simulink model "plantMRUE2"  (R2023b)
settings: Solver=VariableStepAuto  StartTime=0.0  StopTime=7  RelTol=1e-3
model workspace (MATLAB code in the model file):
  | %% True Parameters
  | % Masses
  | mw=0.1;
  | mb=1;
  | M=1.2;
  | 
  | % Distances
  | rho=0.07;
  | l=0.02;
  | d=0.015; % distance A-C
  | 
  | % Electriques
  | L=1e-3;
  | R=1e-1;
  | % r;
  | 
  | % Couples
  | k=1e-2;
  | % alpha=34.6;
  | % beta=2.06e5;
  | 
  | % Moments inertie
  | Iwy=2.45e-4;
  | Ipsi=1.53e-2;
  | 
  | % Utilitaire
  | beta = (M + 2*Iwy/rho^2);
  | gamma = Ipsi + mb*d^2;
  | 
  | %% Nominal Equilibrium Trajectory: Horizontal MRU
  | 
  | % We command speed
  | uref = 1; %m/s
  | psiref = 0;
  | 
  | Usbar = min([2*k/rho*uref; 12]); % should not be >12V
  | 
  | Urbar = Usbar/2; %right
  | Ulbar = Usbar/2;
  | 
  | pbar = 0; % is not in state function, any value fits
  | % normally, should equals ubar*t.
  | ubar = uref;
  | psibar = psiref;
  | vbar = 0;
  | irbar = 0;
  | ilbar = 0;
  | xbar = pbar;
  | ybar = 0;
  | 
  | % IMPORTANT: following only true at t=0s.
  | statebar = [pbar; ubar; psibar; vbar; irbar; ilbar; xbar; ybar];
settings Model: Creator=Jules  LastModifiedBy=Jules

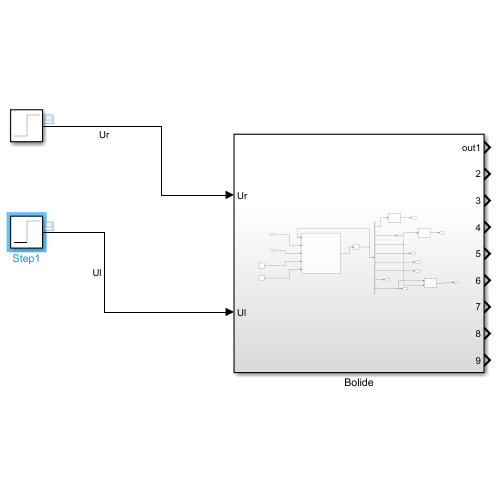
[thumbnail: Simulink's stored preview of the top-level diagram]
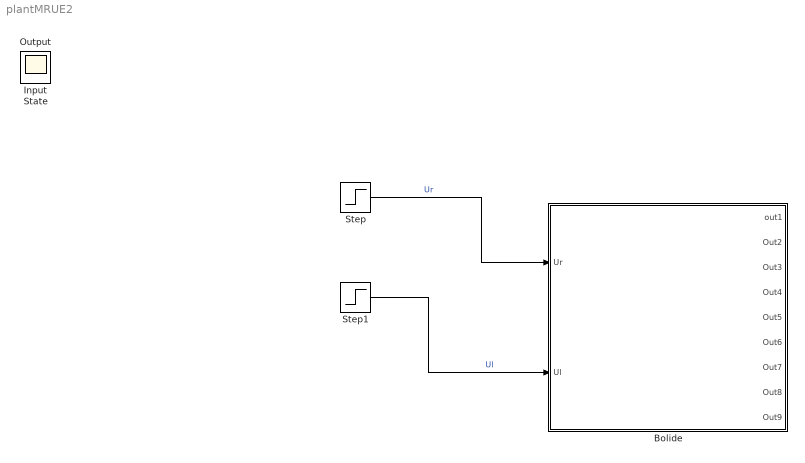
== system plantMRUE2 ==
  Bolide : Subsystem
  Step : Step  Time=5  Before=Urbar  After=Urbar  SampleTime=0
  Step1 : Step  Time=2  Before=Ulbar  After=Ulbar  SampleTime=0
  Input : Scope
  Output : Scope
  State : Scope
  wires:
  Step/1 -> Bolide/1(Ur)  "Ur"
  Step1/1 -> Bolide/2(Ul)  "Ul"

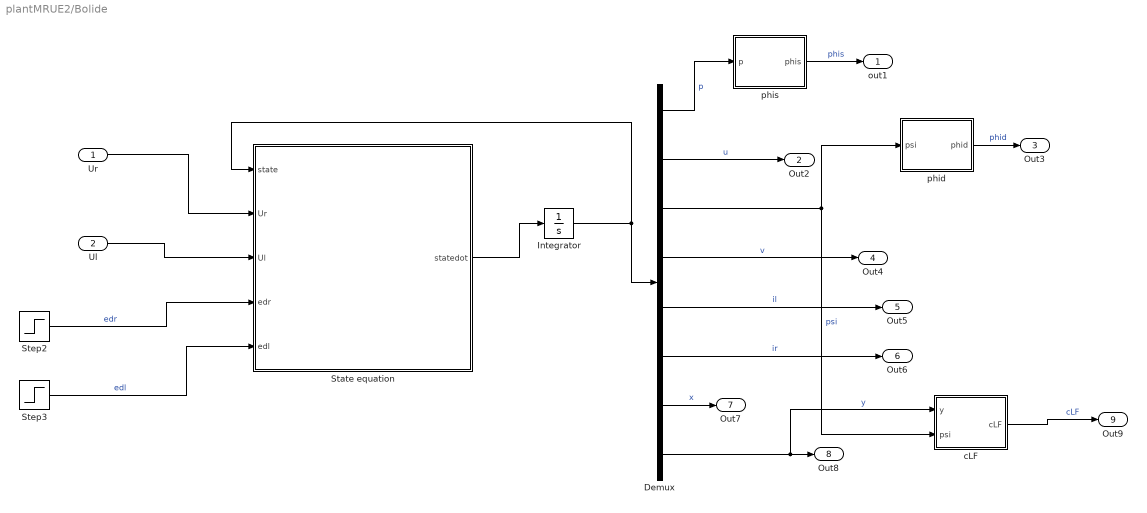
== system plantMRUE2/Bolide ==
  Ur : Inport
  Ul : Inport  Port=2
  Demux : Demux  Outputs=8
  Integrator : Integrator  InitialCondition=statebar
  State equation : MATLAB Function  TreatAsAtomicUnit=on
  Step2 : Step  After=0  SampleTime=0
  Step3 : Step  After=0  SampleTime=0
  cLF : MATLAB Function  TreatAsAtomicUnit=on
  phid : MATLAB Function  TreatAsAtomicUnit=on
  phis : MATLAB Function  TreatAsAtomicUnit=on
  out1 : Outport
  Out2 : Outport  Port=2
  Out3 : Outport  Port=3
  Out4 : Outport  Port=4
  Out5 : Outport  Port=5
  Out6 : Outport  Port=6
  Out7 : Outport  Port=7
  Out8 : Outport  Port=8
  Out9 : Outport  Port=9
  wires:
  Step3/1 -> State equation/5(edl)  "edl"
  State equation/1(statedot) -> Integrator/1
  Integrator/1 -> State equation/1(state), Demux/1
  Step2/1 -> State equation/4(edr)  "edr"
  Ul/1 -> State equation/3(Ul)
  Ur/1 -> State equation/2(Ur)
  Demux/1 -> phis/1(p)  "p"
  Demux/8 -> cLF/1(y), Out8/1  "y"
  Demux/7 -> Out7/1  "x"
  Demux/2 -> Out2/1  "u"
  Demux/6 -> Out6/1  "ir"
  Demux/4 -> Out4/1  "v"
  Demux/5 -> Out5/1  "il"
  phis/1(phis) -> out1/1  "phis"
  Demux/3 -> phid/1(psi), cLF/2(psi)  "psi"
  phid/1(phid) -> Out3/1  "phid"
  cLF/1(cLF) -> Out9/1  "cLF"

== matlab function plantMRUE2/Bolide/cLF ==
  data: y input; cLF output; psi input; psibar parameter; ybar parameter
function cLF = fcn(y, psi, psibar, ybar)

cLF = y/cos(psi - psibar);

== matlab function plantMRUE2/Bolide/State equation ==
  data: state input; statedot output; Ur input; Ul input; edr input; edl input; M parameter; rho parameter; l parameter; Iwy parameter; Ipsi parameter; d parameter; L parameter; R parameter; k parameter; mb parameter; beta parameter; gamma parameter
function statedot = fcn(state,Ur, Ul, edr, edl, M, rho, l, Iwy, Ipsi, d, L, R, k, mb, beta, gamma)
% ed est l'entrée de perturbation, != d (distance AC)
% Model parameters M,Ipsi,d,L,R,k defined in "Model Explorer/Matlab Code"

p = state(1); % intégrale temporelle de u, distance parcourue
u = state(2);
psi = state(3);
v = state(4); % psidot
ir = state(5); % Intensité à gauche
il = state(6);
x = state(7); % ordonnée point A
y = state(8); % abscisse point A

is = ir + il; % Somme
id = ir - il; % Diff
Us = Ur + Ul + edr + edl;
Ud = Ur - Ul + edr - edl;

pdot = u;
udot = 1/beta*(k/rho*is - mb*d*v^2);
psidot = v;
vdot = 1/gamma*(l*k/(2*rho)*id + mb*d*u*v);
isdot = 1/L*(Us - R*is - 2*k/rho*u);
iddot = 1/L*(Ud - R*id - k*l/rho*v);
xdot = cos(psi)*u;
ydot = sin(psi)*u;

irdot = 0.5*(isdot + iddot); % droite
ildot = 0.5*(isdot - iddot);

statedot = [pdot; udot; psidot; vdot; irdot; ildot; xdot; ydot];

== matlab function plantMRUE2/Bolide/phid ==
  data: psi input; phid output; rho parameter; l parameter
function phid = fcn(psi, rho, l)

phid = l/rho*psi;

== matlab function plantMRUE2/Bolide/phis ==
  data: rho parameter; p input; phis output
function phis = fcn(rho,p)

phis = 2/rho*p;
